simulink model "Latero_dir_control"  (R2016a)
settings: Solver=VariableStepAuto  StartTime=0.0  StopTime=20  RelTol=1e-3
values from neighbouring files (symbols this model uses):
  A2 = [Y_beta/U_1 Y_p/U_1 Y_r/U_1-1 g*cos(theta_1)/U_1 ... (first row only)    [Cesna182_flight_dy.m]
  B2 = [Y_da/U_1 Y_dr/U_1 ... (first row only)    [Cesna182_flight_dy.m]
  C2 = [1 0 0 0 ... (first row only)    [Cesna182_flight_dy.m]
  Cc = [0 0 0 0 1]    [Cesna182_flight_dy.m]
  D2 = [0 0 ... (first row only)    [Cesna182_flight_dy.m]
  K1 = K(:,1)    [Cesna182_flight_dy.m]
  Kx = K(:,2:end)    [Cesna182_flight_dy.m]
settings Model: Creator=-F.Machini  LastModifiedBy=-F.Machini

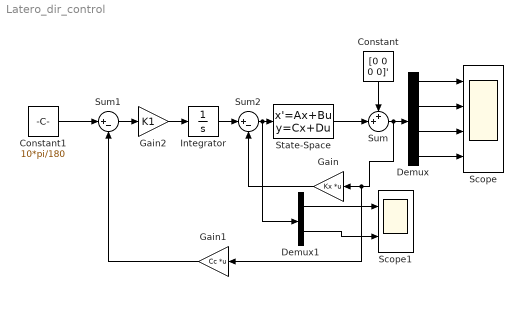
== system Latero_dir_control ==
  Constant : Constant  Value=[0 0 0 0]'
  Constant1 : Constant  Value=10*pi/180
  Demux : Demux
  Demux1 : Demux  Outputs=2
  Gain : Gain  Gain=Kx  Multiplication=Matrix(K*u)
  Gain1 : Gain  Gain=Cc  Multiplication=Matrix(K*u)
  Gain2 : Gain  Gain=K1
  Integrator : Integrator
  Scope : Scope  NumInputPorts=4
  Scope1 : Scope  NumInputPorts=2
  State-Space : StateSpace  A=A2  B=B2  C=C2  D=D2  X0=[0 0 0 0]
  Sum : Sum  Inputs=++|
  Sum1 : Sum  Inputs=|+-
  Sum2 : Sum  Inputs=|+-
  wires:
  Gain/1 -> Sum2/2
  Demux/1 -> Scope/1
  Demux/2 -> Scope/2
  Demux/3 -> Scope/3
  Demux/4 -> Scope/4
  Demux1/1 -> Scope1/1
  Demux1/2 -> Scope1/2
  Sum/1 -> Gain1/1, Gain/1, Demux/1
  Constant/1 -> Sum/1
  State-Space/1 -> Sum/2
  Constant1/1 -> Sum1/1
  Gain1/1 -> Sum1/2
  Sum1/1 -> Gain2/1
  Gain2/1 -> Integrator/1
  Integrator/1 -> Sum2/1
  Sum2/1 -> Demux1/1, State-Space/1
